simulink library "csu_tcm_thruster_command_metering_mtv_ib"  (R2014b)
settings: Solver=ode45  StartTime=0.0  StopTime=10.0  RelTol=1e-3
undefined symbols (not defined in the file or in its folder): act_full_on_duration
libraries: simulink x1, util_info_lib x1, util_common_lib x1
settings Model: Creator=escrane  LastModifiedBy=mstewart

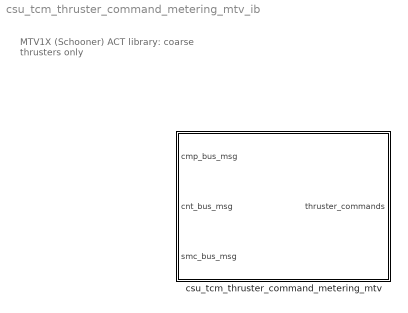
== system csu_tcm_thruster_command_metering_mtv_ib ==
  note: MTV1X (Schooner) ACT library:
      | coarse thrusters only
  csu_tcm_thruster_command_metering_mtv : Subsystem

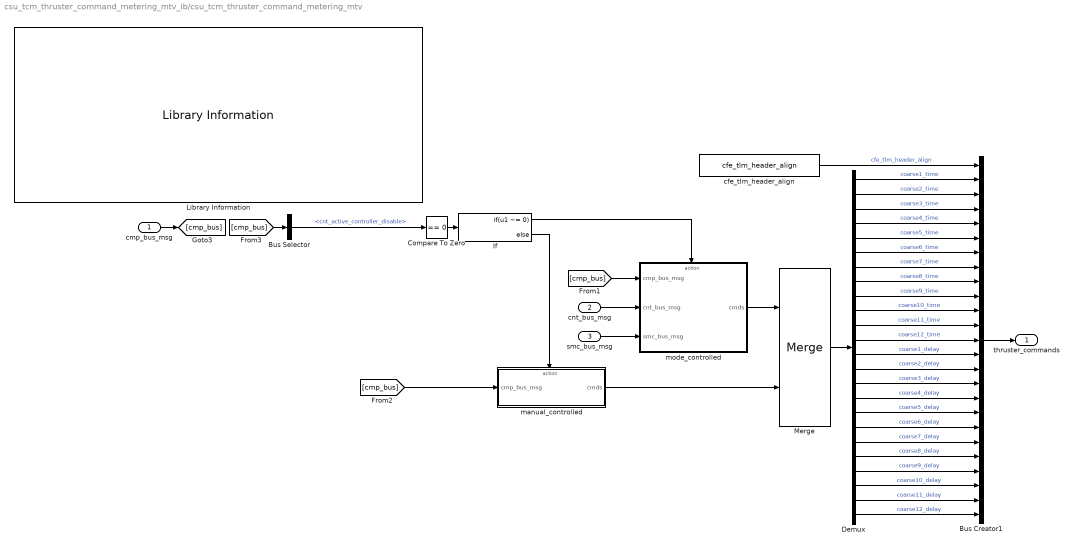
== system csu_tcm_thruster_command_metering_mtv_ib/csu_tcm_thruster_command_metering_mtv ==
  cmp_bus_msg : Inport
  cnt_bus_msg : Inport  Port=2
  smc_bus_msg : Inport  Port=3
  Bus Creator1 : BusCreator  Inputs=25
  Bus Selector : BusSelector  OutputSignals=cnt_active_controller_disable
  Compare To Zero : simulink/Logic and Bit Operations/Compare To Zero  relop===  OutDataTypeStr=boolean
  Demux : Demux  Outputs=24
  If : If  IfExpression=u1 ~= 0
  Library Information : util_info_lib/Library Information  owner='escrane'
  Merge : Merge
  cfe_tlm_header_align : util_common_lib/cfe_tlm_header_align
  manual_controlled : Subsystem  TreatAsAtomicUnit=on
  mode_controlled : Subsystem  TreatAsAtomicUnit=on
  thruster_commands : Outport
  wires:
  Merge/1 -> Demux/1
  Bus Creator1/1 -> thruster_commands/1
  Demux/4 -> Bus Creator1/5  "coarse4_time"
  cfe_tlm_header_align/1 -> Bus Creator1/1  "cfe_tlm_header_align"
  Demux/1 -> Bus Creator1/2  "coarse1_time"
  Demux/8 -> Bus Creator1/9  "coarse8_time"
  Demux/9 -> Bus Creator1/10  "coarse9_time"
  Demux/12 -> Bus Creator1/13  "coarse12_time"
  Demux/7 -> Bus Creator1/8  "coarse7_time"
  Demux/6 -> Bus Creator1/7  "coarse6_time"
  Demux/3 -> Bus Creator1/4  "coarse3_time"
  Demux/5 -> Bus Creator1/6  "coarse5_time"
  Demux/10 -> Bus Creator1/11  "coarse10_time"
  Demux/2 -> Bus Creator1/3  "coarse2_time"
  Demux/11 -> Bus Creator1/12  "coarse11_time"
  Demux/15 -> Bus Creator1/16  "coarse3_delay"
  Demux/16 -> Bus Creator1/17  "coarse4_delay"
  Demux/18 -> Bus Creator1/19  "coarse6_delay"
  Demux/20 -> Bus Creator1/21  "coarse8_delay"
  Demux/14 -> Bus Creator1/15  "coarse2_delay"
  Demux/24 -> Bus Creator1/25  "coarse12_delay"
  Demux/21 -> Bus Creator1/22  "coarse9_delay"
  Demux/17 -> Bus Creator1/18  "coarse5_delay"
  Demux/13 -> Bus Creator1/14  "coarse1_delay"
  Demux/23 -> Bus Creator1/24  "coarse11_delay"
  Demux/19 -> Bus Creator1/20  "coarse7_delay"
  Demux/22 -> Bus Creator1/23  "coarse10_delay"
  [cmp_bus] -> manual_controlled/1(cmp_bus_msg)
  If/2 -> manual_controlled/Action
  If/1 -> mode_controlled/Action
  Compare To Zero/1 -> If/1
  [cmp_bus] -> mode_controlled/1(cmp_bus_msg)
  cnt_bus_msg/1 -> mode_controlled/2(cnt_bus_msg)
  smc_bus_msg/1 -> mode_controlled/3(smc_bus_msg)
  [cmp_bus] -> Bus Selector/1
  cmp_bus_msg/1 -> [cmp_bus]
  manual_controlled/1(cmds) -> Merge/2
  mode_controlled/1(cmds) -> Merge/1
  Bus Selector/1 -> Compare To Zero/1  "<cnt_active_controller_disable>"

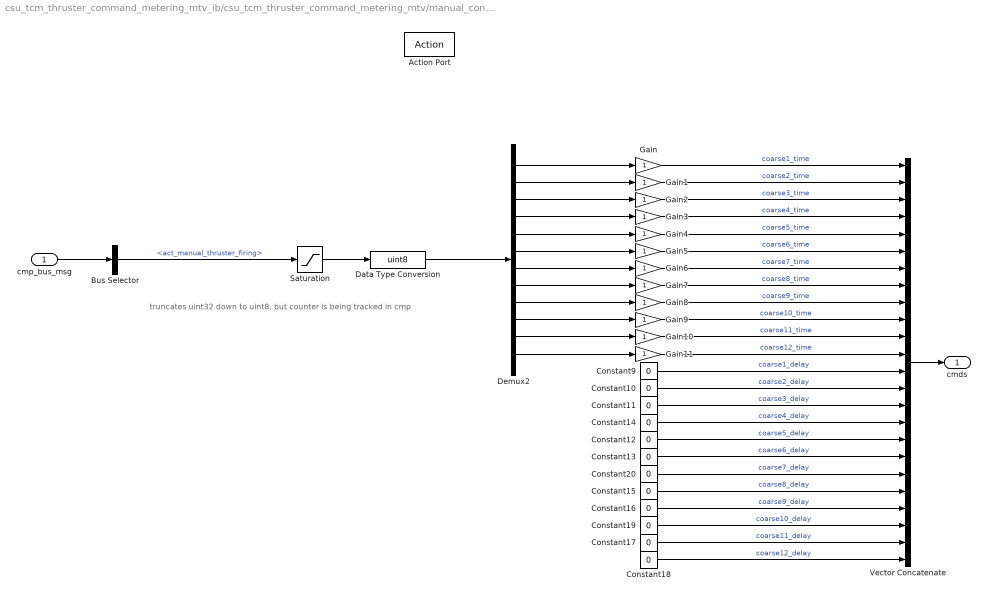
== system csu_tcm_thruster_command_metering_mtv_ib/csu_tcm_thruster_command_metering_mtv/manual_controlled ==
  note: truncates uint32 down to uint8, but counter is being tracked in cmp
  cmp_bus_msg : Inport
  Action Port : ActionPort
  Bus Selector : BusSelector  OutputSignals=act_manual_thruster_firing
  Constant{9..20} (12 alike) : Constant  Value=0  OutDataTypeStr=uint8
  Data Type Conversion : DataTypeConversion  OutDataTypeStr=uint8
  Demux2 : Demux  Outputs=12
  Gain{,1..11} (12 alike) : Gain  OutDataTypeStr=uint8
  Saturation : Saturate  UpperLimit=act_full_on_duration  LowerLimit=0
  Vector Concatenate : Concatenate  NumInputs=24
  cmds : Outport  InitialOutput=zeros(24,1)
  wires:
  Vector Concatenate/1 -> cmds/1
  Gain4/1 -> Vector Concatenate/5  "coarse5_time"
  Gain1/1 -> Vector Concatenate/2  "coarse2_time"
  Gain11/1 -> Vector Concatenate/12  "coarse12_time"
  Gain10/1 -> Vector Concatenate/11  "coarse11_time"
  Gain3/1 -> Vector Concatenate/4  "coarse4_time"
  Gain2/1 -> Vector Concatenate/3  "coarse3_time"
  Gain9/1 -> Vector Concatenate/10  "coarse10_time"
  Gain6/1 -> Vector Concatenate/7  "coarse7_time"
  Gain5/1 -> Vector Concatenate/6  "coarse6_time"
  Gain/1 -> Vector Concatenate/1  "coarse1_time"
  Gain8/1 -> Vector Concatenate/9  "coarse9_time"
  Gain7/1 -> Vector Concatenate/8  "coarse8_time"
  Data Type Conversion/1 -> Demux2/1
  Demux2/1 -> Gain/1
  Demux2/2 -> Gain1/1
  Demux2/3 -> Gain2/1
  Demux2/4 -> Gain3/1
  Demux2/5 -> Gain4/1
  Demux2/6 -> Gain5/1
  Demux2/12 -> Gain11/1
  Demux2/11 -> Gain10/1
  Demux2/10 -> Gain9/1
  Demux2/9 -> Gain8/1
  Demux2/8 -> Gain7/1
  Demux2/7 -> Gain6/1
  Bus Selector/1 -> Saturation/1  "<act_manual_thruster_firing>"
  cmp_bus_msg/1 -> Bus Selector/1
  Constant11/1 -> Vector Concatenate/15  "coarse3_delay"
  Constant14/1 -> Vector Concatenate/16  "coarse4_delay"
  Constant13/1 -> Vector Concatenate/18  "coarse6_delay"
  Constant15/1 -> Vector Concatenate/20  "coarse8_delay"
  Constant10/1 -> Vector Concatenate/14  "coarse2_delay"
  Constant18/1 -> Vector Concatenate/24  "coarse12_delay"
  Constant16/1 -> Vector Concatenate/21  "coarse9_delay"
  Constant12/1 -> Vector Concatenate/17  "coarse5_delay"
  Constant9/1 -> Vector Concatenate/13  "coarse1_delay"
  Constant17/1 -> Vector Concatenate/23  "coarse11_delay"
  Constant20/1 -> Vector Concatenate/19  "coarse7_delay"
  Constant19/1 -> Vector Concatenate/22  "coarse10_delay"
  Saturation/1 -> Data Type Conversion/1

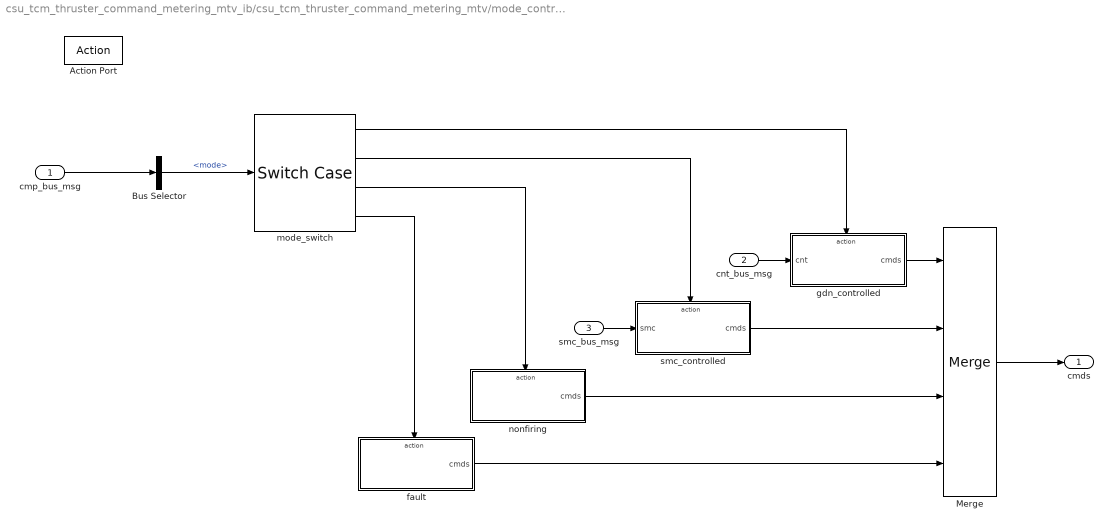
== system csu_tcm_thruster_command_metering_mtv_ib/csu_tcm_thruster_command_metering_mtv/mode_controlled ==
  cmp_bus_msg : Inport
  cnt_bus_msg : Inport  Port=2
  smc_bus_msg : Inport  Port=3
  Action Port : ActionPort
  Bus Selector : BusSelector  OutputSignals=mode
  Merge : Merge  Inputs=4
  fault : Subsystem  TreatAsAtomicUnit=on
  gdn_controlled : Subsystem  TreatAsAtomicUnit=on
  mode_switch : SwitchCase  CaseConditions={ [uint8(enum_mode.pointing), uint8(enum_mode.deltav), uint8(enum_mode.deorbit), uint8(enum_mode.braking) uint8(enum_mode.landing)], uint8(enum_mode.safe), [uint8(enum_mode.startup), uint8(enum_mode.surface), uint8(enum_mode.safesurface)]}
  nonfiring : Subsystem  TreatAsAtomicUnit=on
  smc_controlled : Subsystem  TreatAsAtomicUnit=on
  cmds : Outport  InitialOutput=zeros(24,1)
  wires:
  cmp_bus_msg/1 -> Bus Selector/1
  fault/1(cmds) -> Merge/4
  mode_switch/4 -> fault/Action
  Merge/1 -> cmds/1
  smc_bus_msg/1 -> smc_controlled/1(smc)
  nonfiring/1(cmds) -> Merge/3
  smc_controlled/1(cmds) -> Merge/2
  gdn_controlled/1(cmds) -> Merge/1
  mode_switch/3 -> nonfiring/Action
  mode_switch/2 -> smc_controlled/Action
  mode_switch/1 -> gdn_controlled/Action
  cnt_bus_msg/1 -> gdn_controlled/1(cnt)
  Bus Selector/1 -> mode_switch/1  "<mode>"

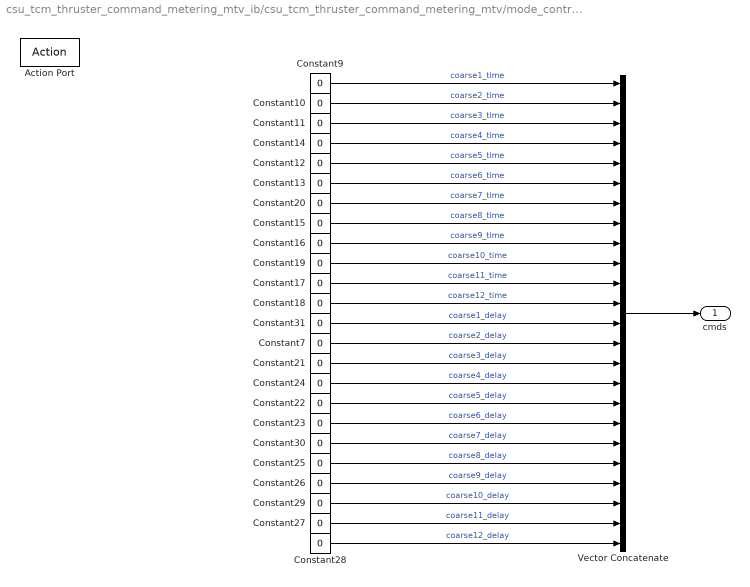
== system csu_tcm_thruster_command_metering_mtv_ib/csu_tcm_thruster_command_metering_mtv/mode_controlled/fault ==
  Action Port : ActionPort
  Constant{7,9..31} (24 alike) : Constant  Value=0  OutDataTypeStr=uint8
  Vector Concatenate : Concatenate  NumInputs=24
  cmds : Outport  InitialOutput=zeros(24,1)
  wires:
  Vector Concatenate/1 -> cmds/1
  Constant9/1 -> Vector Concatenate/1  "coarse1_time"
  Constant15/1 -> Vector Concatenate/8  "coarse8_time"
  Constant16/1 -> Vector Concatenate/9  "coarse9_time"
  Constant18/1 -> Vector Concatenate/12  "coarse12_time"
  Constant20/1 -> Vector Concatenate/7  "coarse7_time"
  Constant14/1 -> Vector Concatenate/4  "coarse4_time"
  Constant13/1 -> Vector Concatenate/6  "coarse6_time"
  Constant11/1 -> Vector Concatenate/3  "coarse3_time"
  Constant12/1 -> Vector Concatenate/5  "coarse5_time"
  Constant19/1 -> Vector Concatenate/10  "coarse10_time"
  Constant10/1 -> Vector Concatenate/2  "coarse2_time"
  Constant17/1 -> Vector Concatenate/11  "coarse11_time"
  Constant21/1 -> Vector Concatenate/15  "coarse3_delay"
  Constant24/1 -> Vector Concatenate/16  "coarse4_delay"
  Constant23/1 -> Vector Concatenate/18  "coarse6_delay"
  Constant25/1 -> Vector Concatenate/20  "coarse8_delay"
  Constant7/1 -> Vector Concatenate/14  "coarse2_delay"
  Constant28/1 -> Vector Concatenate/24  "coarse12_delay"
  Constant26/1 -> Vector Concatenate/21  "coarse9_delay"
  Constant22/1 -> Vector Concatenate/17  "coarse5_delay"
  Constant31/1 -> Vector Concatenate/13  "coarse1_delay"
  Constant27/1 -> Vector Concatenate/23  "coarse11_delay"
  Constant30/1 -> Vector Concatenate/19  "coarse7_delay"
  Constant29/1 -> Vector Concatenate/22  "coarse10_delay"

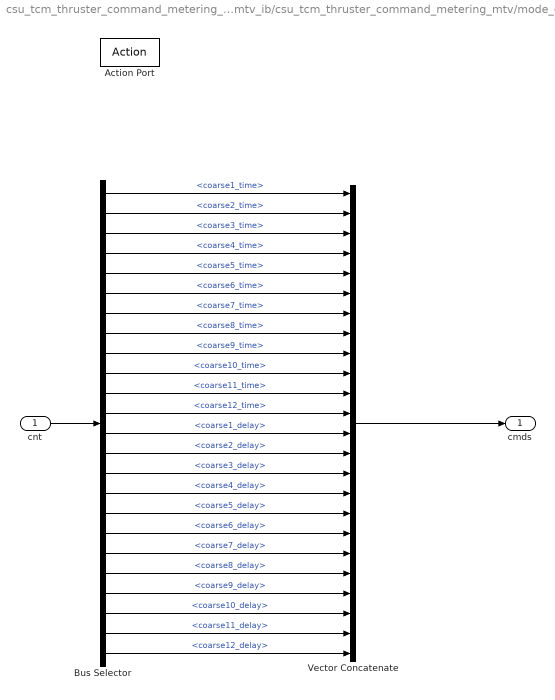
== system csu_tcm_thruster_command_metering_mtv_ib/csu_tcm_thruster_command_metering_mtv/mode_controlled/gdn_controlled ==
  cnt : Inport
  Action Port : ActionPort
  Bus Selector : BusSelector  OutputSignals=coarse1_time,coarse2_time,coarse3_time,coarse4_time,coarse5_time,coarse6_time,coarse7_time,coarse8_time,coarse9_time,coarse10_time,coarse11_time,coarse12_time,coarse1_delay,coarse2_delay,coarse3_delay,coarse4_delay,coarse5_delay,coarse6_delay,coarse7_delay,coarse8_delay,coarse9_delay,coarse10_delay,coarse11_delay,coarse12_delay
  Vector Concatenate : Concatenate  NumInputs=24
  cmds : Outport  InitialOutput=zeros(24,1)
  wires:
  Vector Concatenate/1 -> cmds/1
  Bus Selector/2 -> Vector Concatenate/2  "<coarse2_time>"
  Bus Selector/6 -> Vector Concatenate/6  "<coarse6_time>"
  Bus Selector/17 -> Vector Concatenate/17  "<coarse5_delay>"
  Bus Selector/16 -> Vector Concatenate/16  "<coarse4_delay>"
  Bus Selector/10 -> Vector Concatenate/10  "<coarse10_time>"
  Bus Selector/9 -> Vector Concatenate/9  "<coarse9_time>"
  Bus Selector/8 -> Vector Concatenate/8  "<coarse8_time>"
  Bus Selector/12 -> Vector Concatenate/12  "<coarse12_time>"
  Bus Selector/20 -> Vector Concatenate/20  "<coarse8_delay>"
  Bus Selector/5 -> Vector Concatenate/5  "<coarse5_time>"
  Bus Selector/23 -> Vector Concatenate/23  "<coarse11_delay>"
  Bus Selector/3 -> Vector Concatenate/3  "<coarse3_time>"
  Bus Selector/11 -> Vector Concatenate/11  "<coarse11_time>"
  Bus Selector/22 -> Vector Concatenate/22  "<coarse10_delay>"
  Bus Selector/21 -> Vector Concatenate/21  "<coarse9_delay>"
  Bus Selector/19 -> Vector Concatenate/19  "<coarse7_delay>"
  Bus Selector/15 -> Vector Concatenate/15  "<coarse3_delay>"
  Bus Selector/4 -> Vector Concatenate/4  "<coarse4_time>"
  Bus Selector/7 -> Vector Concatenate/7  "<coarse7_time>"
  Bus Selector/18 -> Vector Concatenate/18  "<coarse6_delay>"
  Bus Selector/1 -> Vector Concatenate/1  "<coarse1_time>"
  Bus Selector/24 -> Vector Concatenate/24  "<coarse12_delay>"
  Bus Selector/13 -> Vector Concatenate/13  "<coarse1_delay>"
  Bus Selector/14 -> Vector Concatenate/14  "<coarse2_delay>"
  cnt/1 -> Bus Selector/1

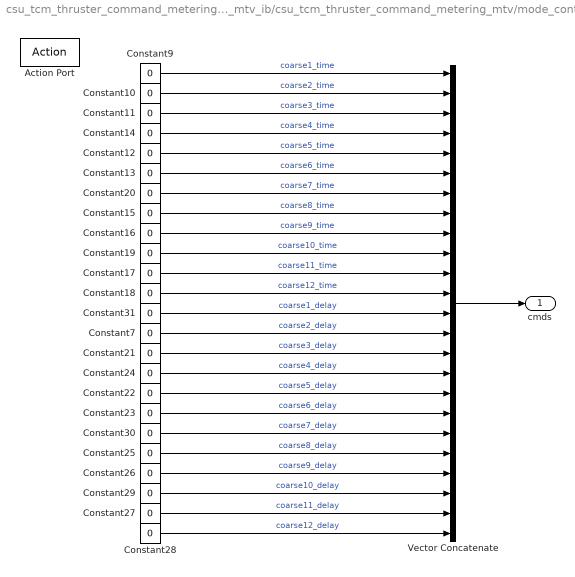
== system csu_tcm_thruster_command_metering_mtv_ib/csu_tcm_thruster_command_metering_mtv/mode_controlled/nonfiring ==
  Action Port : ActionPort
  Constant{7,9..31} (24 alike) : Constant  Value=0  OutDataTypeStr=uint8
  Vector Concatenate : Concatenate  NumInputs=24
  cmds : Outport  InitialOutput=zeros(24,1)
  wires:
  Vector Concatenate/1 -> cmds/1
  Constant9/1 -> Vector Concatenate/1  "coarse1_time"
  Constant15/1 -> Vector Concatenate/8  "coarse8_time"
  Constant16/1 -> Vector Concatenate/9  "coarse9_time"
  Constant18/1 -> Vector Concatenate/12  "coarse12_time"
  Constant20/1 -> Vector Concatenate/7  "coarse7_time"
  Constant14/1 -> Vector Concatenate/4  "coarse4_time"
  Constant13/1 -> Vector Concatenate/6  "coarse6_time"
  Constant11/1 -> Vector Concatenate/3  "coarse3_time"
  Constant12/1 -> Vector Concatenate/5  "coarse5_time"
  Constant19/1 -> Vector Concatenate/10  "coarse10_time"
  Constant10/1 -> Vector Concatenate/2  "coarse2_time"
  Constant17/1 -> Vector Concatenate/11  "coarse11_time"
  Constant21/1 -> Vector Concatenate/15  "coarse3_delay"
  Constant24/1 -> Vector Concatenate/16  "coarse4_delay"
  Constant23/1 -> Vector Concatenate/18  "coarse6_delay"
  Constant25/1 -> Vector Concatenate/20  "coarse8_delay"
  Constant7/1 -> Vector Concatenate/14  "coarse2_delay"
  Constant28/1 -> Vector Concatenate/24  "coarse12_delay"
  Constant26/1 -> Vector Concatenate/21  "coarse9_delay"
  Constant22/1 -> Vector Concatenate/17  "coarse5_delay"
  Constant31/1 -> Vector Concatenate/13  "coarse1_delay"
  Constant27/1 -> Vector Concatenate/23  "coarse11_delay"
  Constant30/1 -> Vector Concatenate/19  "coarse7_delay"
  Constant29/1 -> Vector Concatenate/22  "coarse10_delay"

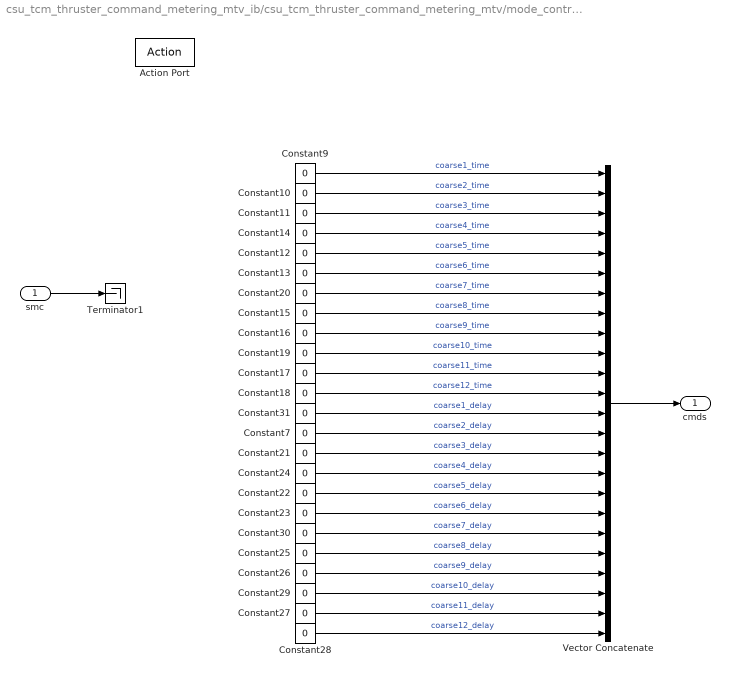
== system csu_tcm_thruster_command_metering_mtv_ib/csu_tcm_thruster_command_metering_mtv/mode_controlled/smc_controlled ==
  smc : Inport
  Action Port : ActionPort
  Constant{7,9..31} (24 alike) : Constant  Value=0  OutDataTypeStr=uint8
  Terminator1 : Terminator
  Vector Concatenate : Concatenate  NumInputs=24
  cmds : Outport  InitialOutput=zeros(24,1)
  wires:
  Vector Concatenate/1 -> cmds/1
  Constant9/1 -> Vector Concatenate/1  "coarse1_time"
  Constant15/1 -> Vector Concatenate/8  "coarse8_time"
  Constant16/1 -> Vector Concatenate/9  "coarse9_time"
  Constant18/1 -> Vector Concatenate/12  "coarse12_time"
  Constant20/1 -> Vector Concatenate/7  "coarse7_time"
  Constant14/1 -> Vector Concatenate/4  "coarse4_time"
  Constant13/1 -> Vector Concatenate/6  "coarse6_time"
  Constant11/1 -> Vector Concatenate/3  "coarse3_time"
  Constant12/1 -> Vector Concatenate/5  "coarse5_time"
  Constant19/1 -> Vector Concatenate/10  "coarse10_time"
  Constant10/1 -> Vector Concatenate/2  "coarse2_time"
  Constant17/1 -> Vector Concatenate/11  "coarse11_time"
  Constant21/1 -> Vector Concatenate/15  "coarse3_delay"
  Constant24/1 -> Vector Concatenate/16  "coarse4_delay"
  Constant23/1 -> Vector Concatenate/18  "coarse6_delay"
  Constant25/1 -> Vector Concatenate/20  "coarse8_delay"
  Constant7/1 -> Vector Concatenate/14  "coarse2_delay"
  Constant28/1 -> Vector Concatenate/24  "coarse12_delay"
  Constant26/1 -> Vector Concatenate/21  "coarse9_delay"
  Constant22/1 -> Vector Concatenate/17  "coarse5_delay"
  Constant31/1 -> Vector Concatenate/13  "coarse1_delay"
  Constant27/1 -> Vector Concatenate/23  "coarse11_delay"
  Constant30/1 -> Vector Concatenate/19  "coarse7_delay"
  Constant29/1 -> Vector Concatenate/22  "coarse10_delay"
  smc/1 -> Terminator1/1
